simulink model "b0307"  (R2025b)
settings: Solver=ode4  StartTime=0.0  StopTime=533  FixedStep=0.001  RelTol=1e-3
values from neighbouring files (symbols this model uses):
  alpha_vector = [-8 -4 -2 0 2 3 4 5 6 8 10 12]    [aerodata.mat]    (also in airdate.m = [-8 -4 -2 0 2 3 4 5 6 8 10 12]')
  alpha_vector1 = [-4 0 4 8]    [aerodata.mat]    (also in airdate.m = [-4, 0, 4, 8])
  alpha_vector2 = [-4 0 4 8]    [aerodata.mat]    (also in airdate.m = [-4, 0, 4, 8])
  b_ref = 2.24    [init.m]
  beta_vector1 = [-8 -4 0 4 8]    [aerodata.mat]    (also in airdate.m = [-8, -4, 0, 4, 8])
  c_ref = 0.165    [init.m]
  CD_alpha = [0.0485620740363 0.0318356514345 0.0317790643102 0.0364045204537 0.0445214008185 0.0513240541996 0.0580305477533 0.0657045426134 0.0744839493029 0.0955551011208 0.133141813384 0.18014601666]    [aerodata.mat]    (also in airdate.m = alpha_matrix(1:length(alpha_vector), 3))
  CD_beta = [0.0413061898506 0.0345389961433 0.0318356514345 0.0345389961433 0.0413061898506 0.0436826 0.0385768 0.0364045204537 0.0371657170379 0.0408604078007 0.0616785 0.0590205 ... (20 elements, 5x4)]    [aerodata.mat]    (also in airdate.m = reshape(beta_matrix(:, 3), [n_beta, n_alpha1]))
  CD_ELE = [0.0367807192259 0.0308673912055 0.0306770192219 0.0329799710874 0.0376266798938 0.0362372767671 0.0347486720958 0.0364045204537 0.0395900797854 0.0493584368547 0.0520155680915 0.0546030505455 ... (20 elements, 5x4)]    [aerodata.mat]    (also in airdate.m = reshape(def_ELE_L_matrix(:, 4), [n_ele, n_alpha2]))
  CL_alpha = [-0.316928256932 -0.0246785813034 0.130283368141 0.288945629191 0.449323999783 0.525648685194 0.60297649153 0.678148219772 0.750129216407 0.872962476804 0.920788454091 0.929116005788]    [aerodata.mat]    (also in airdate.m = alpha_matrix(1:length(alpha_vector), 5))
  Cl_alpha = [-0.000640872979326 1.08116418077e-05 2.92649499784e-07 0 -0.000437066219056 -0.000762440123061 -0.000973039479867 -0.00125684277681 -0.00152984821199 -0.00187186802219 -0.00184918573213 0.00105936824418]    [aerodata.mat]    (also in airdate.m = alpha_matrix(1:length(alpha_vector), 6))
  CL_beta = [-0.0254603323809 -0.0249297140554 -0.0246785813034 -0.0249297140554 -0.0254603323809 0.27807 0.286078 0.288945629191 0.286671909097 0.27925707766 0.602944 0.604359 ... (20 elements, 5x4)]    [aerodata.mat]    (also in airdate.m = reshape(beta_matrix(:, 5), [n_beta, n_alpha1]))
  Cl_beta = [0.000236297001567 0.000139283426539 1.08116418077e-05 -0.000139283426539 -0.000236297001567 0.000738099 0.000299952 -0.000269027677603 -0.00096883985561 -0.00179948469019 0.0018278 0.000411742 ... (20 elements, 5x4)]    [aerodata.mat]    (also in airdate.m = reshape(beta_matrix(:, 6), [n_beta, n_alpha1]))
  CL_ELE = [-0.209245674304 -0.118097376915 -0.0691301102129 -0.0258480382303 0.0604619193477 0.145712419951 0.241076881119 0.288945629191 0.337037782187 0.427489906586 0.461138992576 0.556875751161 ... (20 elements, 5x4)]    [aerodata.mat]    (also in airdate.m = reshape(def_ELE_L_matrix(:, 6), [n_ele, n_alpha2]))
  Cl_ELE = [-0.0251269797289 -0.008426817179 0.000240167384607 0.00909972758991 0.0243415498089 -0.0265884432031 -0.00914521718395 -0.000269027677603 0.00845228310052 0.0248325485851 -0.027436226674 -0.00980497383292 ... (20 elements, 5x4)]    [aerodata.mat]    (also in airdate.m = reshape(def_ELE_L_matrix(:, 7), [n_ele, n_alpha2]))
  Cl_ELER = [0.0251269797289 0.008426817179 -0.000240167384607 -0.00909972758991 -0.0243415498089 0.0265884432031 0.00914521718395 0.000269027677603 -0.00845228310052 -0.0248325485851 0.027436226674 0.00980497383292 ... (20 elements, 5x4)]    [aerodata.mat]    (also in airdate.m = -Cl_ELE)
  Cm_alpha = [0.0626600725128 0.0530799370217 0.0636683163616 0.0662391704182 0.0712518097577 0.059404297375 0.0463976401398 0.0265816846325 -0.000744425674427 -0.0975303788137 -0.390110677431 -0.549514574144]    [aerodata.mat]    (also in airdate.m = alpha_matrix(1:length(alpha_vector), 7))
  Cm_beta = [0.0443576401398 0.0504624 0.0530799370217 0.0504624 0.0443576401398 0.0399653 0.0540624 0.0662391704182 0.0664956832735 0.054831924477 -0.0180401 0.0135503 ... (20 elements, 5x4)]    [aerodata.mat]    (also in airdate.m = reshape(beta_matrix(:, 7), [n_beta, n_alpha1]))
  Cm_ELE = [0.536255917663 0.147824254744 -0.0380057879786 -0.216266528425 -0.571251073338 0.641418774301 0.260817426469 0.0662391704182 -0.124486673615 -0.489660800762 0.614897515281 0.238355554417 ... (20 elements, 5x4)]    [aerodata.mat]    (also in airdate.m = reshape(def_ELE_L_matrix(:, 8), [n_ele, n_alpha2]))
  Cn_alpha = [-0.000921303455433 -0.000100429360075 -5.32721662229e-05 0 -0.000448050865233 -0.000265660085507 -0.000172455805371 -9.0297395806e-05 0.000114919609077 0.000960640598216 0.000800025371357 0.00296984280205]    [aerodata.mat]    (also in airdate.m = alpha_matrix(1:length(alpha_vector), 8))
  Cn_beta = [-0.0118929295373 -0.00644657732457 -0.000100429360075 0.00644657732457 0.0118929295373 -0.00932594 -0.00455936 -0.000185600362027 0.00379534502079 0.00738347341913 -0.00140779 -0.00161764 ... (20 elements, 5x4)]    [aerodata.mat]    (also in airdate.m = reshape(beta_matrix(:, 8), [n_beta, n_alpha1]))
  Cn_ELE = [-0.000978013358228 0.000374192483935 0.000921206928251 0.00041612460588 -0.00121710528947 -0.00219374024917 -0.000325070715732 -0.000185600362027 -8.6022941264e-05 -0.000494144283219 -0.00293821245405 -0.00054824676514 ... (20 elements, 5x4)]    [aerodata.mat]    (also in airdate.m = reshape(def_ELE_L_matrix(:, 9), [n_ele, n_alpha2]))
  Cn_ELER = [0.000978013358228 -0.000374192483935 -0.000921206928251 -0.00041612460588 0.00121710528947 0.00219374024917 0.000325070715732 0.000185600362027 8.6022941264e-05 0.000494144283219 0.00293821245405 0.00054824676514 ... (20 elements, 5x4)]    [aerodata.mat]    (also in airdate.m = -Cn_ELE)
  CY_alpha = [0.00094331940582 8.91316440807e-05 0.00163191368255 0 0.00399491029065 0.00495876756067 0.00538171092978 0.00589122371949 0.00623993707833 0.00649420059364 0.0115896523304 0.0134657730505]    [aerodata.mat]    (also in airdate.m = alpha_matrix(1:length(alpha_vector), 4))
  CY_beta = [0.0411779977966 0.0260529022214 8.91316440807e-05 -0.0260529022214 -0.0411779977966 0.0626258 0.0323129 0.00352355870293 -0.0237421290295 -0.0494841840717 0.0422501 0.0258494 ... (20 elements, 5x4)]    [aerodata.mat]    (also in airdate.m = reshape(beta_matrix(:, 4), [n_beta, n_alpha1]))
  CY_ELE = [0.00947355235179 0.0032440045221 0.000919743913066 3.31170671791e-05 -0.00246607912146 0.00984559930618 0.00470476147172 0.00352355870293 0.00144187166173 -0.00241087659802 0.0116316527742 0.00697261934365 ... (20 elements, 5x4)]    [aerodata.mat]    (also in airdate.m = reshape(def_ELE_L_matrix(:, 5), [n_ele, n_alpha2]))
  def_ELE_L_vector = [-15 -5 0 5 15]    [aerodata.mat]    (also in airdate.m = [-15, -5, 0, 5, 15])
  delta_max = 15    [init.m]
  fly_pt = [0 397.202504295 825.49541327 510 4564.45331975 4885.85117615 4860 4885.85117615 4899.67498335 5610.29789652 5624.12170371 5880 ... (135 elements, 27x5)]    [baseline_fly_plan.mat]    (also in debug_replay_flyphase.m = evalin('base','fly_pt'); dubins_path_planning.m = dubins.filter_waypoints(fly_pt); fly_planfjy.mat; make_orbit_plan.m = dubins.filter_waypoints(fly_pt))
  g = 9.8    [Astar.m]    (also in dubins_path_planning.m; init.m; make_orbit_plan.m; make_route_plan.m)
  I = [I_x -I_xy -I_xz ... (first row only)    [init.m]
  I_inv = inv(I)    [init.m]
  kal = (wn^2-a_24(3))/(2*zeta*wn)    [controller.m]
  ki = 0.1*kphi    (= 0.75)    [controller.m]
  kn = (-2.2*wn^2*g)/(Tr*(wn^2+a_24(3))*Vc*Z_al)    [controller.m]
  kp = 2*zeta2*wn2/N_delatr_bar    [controller.m]
  kphi = wn2/2/zeta2    (= 7.5)    [controller.m]
  kq = -(2*zeta*wn) / a_25    [controller.m]
  mass = 27.1    [init.m]
  pitch_max = 30    [init.m]
  psi_0 = 0 * (pi/180)    (= 0)    [init.m]
  psi_t = 0    [Astar.m]    (also in init.m)
  roll_max = 30*pi/180    (= 0.523598775598)    [Astar.m]    (also in dubins_path_planning.m = 0.261799387799; init.m = 30)
  S_ref = 0.7    [init.m]
  theta_0 = 30 * (pi/180)    (= 0.523598775598)    [init.m]
  theta_t = 0    [Astar.m]    (also in init.m)
  u_0 = Vc_0*cos(beta_0)*cos(alpha_0)    [init.m]
  v_0 = Vc_0*sin(beta_0)    [init.m]
  V_t = 0    [Astar.m]    (also in init.m)
  Vc = 34    [Astar.m]    (also in dubins_path_planning.m; init.m; make_orbit_plan.m; make_route_plan.m)
  w_0 = Vc_0*cos(beta_0)*sin(alpha_0)    [init.m]
  W_down = 0    [init.m]
  W_east = 0    [init.m]
  W_north = 0    [init.m]
  xt0 = 6500    [Astar.m]    (also in init.m)
  yt0 = 9000    [Astar.m]    (also in init.m)
  Z_al = (CD_alpha(10)+CL_al)*(q_0*S_ref/(mass*Vc))    [controller.m]
  zt0 = 0    [Astar.m]    (also in init.m)
undefined symbols (not defined in the file or in its folder): beta_vector0
libraries: matrix_library x2, simulink x1, aerolibatmos2 x1, slpidlib x1
(part 2 of 2)

== system b0307/气动力和气动力矩/气动力/侧力 ==
  q_p1 : Inport
  beta1 : Inport  Port=2
  alpha1 : Inport  Port=3
  delta_l : Inport  Port=4
  delta_r : Inport  Port=5
  Add : Sum  Inputs=-+
  Add1 : Sum  Inputs=+-
  Add2 : Sum  Inputs=+-
  Add3 : Sum  Inputs=+-
  Add4 : Sum
  Add5 : Sum  Inputs=++++
  CY_alpha : Lookup_n-D  NumberOfTableDimensions=1  BreakpointsForDimension1=alpha_vector  BreakpointsForDimension2=beta_vector0  BreakpointsForDimension3=[5, 7]  Table=CY_alpha  InternalRulePriority=Speed  RndMeth=Simplest
  CY_alpha0 : Lookup_n-D  NumberOfTableDimensions=1  BreakpointsForDimension1=alpha_vector  BreakpointsForDimension2=beta_vector0  BreakpointsForDimension3=[5, 7]  Table=CY_alpha  InternalRulePriority=Speed  RndMeth=Simplest
  CY_beta : Lookup_n-D  BreakpointsForDimension1=beta_vector1  BreakpointsForDimension2=alpha_vector1  BreakpointsForDimension3=[5, 7]  Table=CY_beta  InternalRulePriority=Speed  RndMeth=Simplest
      settings: InputPortMap=u0,u1
  CY_beta0 : Lookup_n-D  BreakpointsForDimension1=beta_vector1  BreakpointsForDimension2=alpha_vector1  BreakpointsForDimension3=[5, 7]  Table=CY_beta  InternalRulePriority=Speed  RndMeth=Simplest
      settings: InputPortMap=u0,u1
  CY_delta_l : Lookup_n-D  BreakpointsForDimension1=def_ELE_L_vector  BreakpointsForDimension2=alpha_vector2  BreakpointsForDimension3=[5, 7]  Table=CY_ELE  InternalRulePriority=Speed  RndMeth=Simplest
      settings: InputPortMap=u0,u1
  CY_delta_l0 : Lookup_n-D  BreakpointsForDimension1=def_ELE_L_vector  BreakpointsForDimension2=alpha_vector2  BreakpointsForDimension3=[5, 7]  Table=CY_ELE  InternalRulePriority=Speed  RndMeth=Simplest
      settings: InputPortMap=u0,u1
  CY_delta_r : Lookup_n-D  BreakpointsForDimension1=def_ELE_L_vector  BreakpointsForDimension2=alpha_vector2  BreakpointsForDimension3=[5, 7]  Table=CY_ELE  InternalRulePriority=Speed  RndMeth=Simplest
      settings: InputPortMap=u0,u1
  CY_delta_r0 : Lookup_n-D  BreakpointsForDimension1=def_ELE_L_vector  BreakpointsForDimension2=alpha_vector2  BreakpointsForDimension3=[5, 7]  Table=CY_ELE  InternalRulePriority=Speed  RndMeth=Simplest
      settings: InputPortMap=u0,u1
  Constant : Constant  Value=0
  Constant1 : Constant  Value=0
  Constant7 : Constant  Value=S_ref
  Product : Product  Inputs=3
  Saturation : Saturate  UpperLimit=8  LowerLimit=-4
  侧力Y : Outport
  wires:
  Add3/1 -> Add4/2
  delta_l/1 -> CY_delta_l/1
  CY_delta_l0/1 -> Add2/2
  Add1/1 -> Add5/3
  CY_alpha/1 -> Add/2
  q_p1/1 -> Product/1
  Add4/1 -> Add5/4
  Constant7/1 -> Product/3
  Add5/1 -> Product/2
  Add2/1 -> Add4/1
  CY_delta_r/1 -> Add3/1
  CY_alpha0/1 -> Add/1, Add5/1
  Add/1 -> Add5/2
  Product/1 -> 侧力Y/1
  CY_beta0/1 -> Add1/2
  Constant1/1 -> CY_delta_r0/1, CY_delta_l0/1
  CY_delta_l/1 -> Add2/1
  Constant/1 -> CY_beta0/1, CY_alpha0/1
  CY_delta_r0/1 -> Add3/2
  delta_r/1 -> CY_delta_r/1
  alpha1/1 -> Saturation/1, CY_alpha/1
  beta1/1 -> CY_beta/1
  CY_beta/1 -> Add1/1
  Saturation/1 -> CY_beta0/2, CY_delta_l/2, CY_delta_l0/2, CY_delta_r0/2, CY_delta_r/2, CY_beta/2

== system b0307/气动力和气动力矩/气动力/升力 ==
  q_p : Inport
  beta : Inport  Port=2
  alpha : Inport  Port=3
  delta_l : Inport  Port=4
  delta_r : Inport  Port=5
  Add : Sum  Inputs=-+
  Add1 : Sum  Inputs=+-
  Add2 : Sum  Inputs=+-
  Add3 : Sum  Inputs=+-
  Add4 : Sum
  Add5 : Sum  Inputs=++++
  CL_alpha : Lookup_n-D  NumberOfTableDimensions=1  BreakpointsForDimension1=alpha_vector  Table=CL_alpha  ExtrapMethod=Clip  UseLastTableValue=on  InternalRulePriority=Speed  RndMeth=Simplest
  CL_beta : Lookup_n-D  BreakpointsForDimension1=beta_vector1  BreakpointsForDimension2=alpha_vector1  BreakpointsForDimension3=[5, 7]  Table=CL_beta  InternalRulePriority=Speed  RndMeth=Simplest
      settings: InputPortMap=u0,u1
  CL_beta0 : Lookup_n-D  BreakpointsForDimension1=beta_vector1  BreakpointsForDimension2=alpha_vector1  BreakpointsForDimension3=[5, 7]  Table=CL_beta  InternalRulePriority=Speed  RndMeth=Simplest
      settings: InputPortMap=u0,u1
  CL_delta_l : Lookup_n-D  BreakpointsForDimension1=def_ELE_L_vector  BreakpointsForDimension2=alpha_vector2  BreakpointsForDimension3=[5, 7]  Table=CL_ELE  InternalRulePriority=Speed  RndMeth=Simplest
      settings: InputPortMap=u0,u1
  CL_delta_l0 : Lookup_n-D  BreakpointsForDimension1=def_ELE_L_vector  BreakpointsForDimension2=alpha_vector2  BreakpointsForDimension3=[5, 7]  Table=CL_ELE  InternalRulePriority=Speed  RndMeth=Simplest
      settings: InputPortMap=u0,u1
  CL_delta_r : Lookup_n-D  BreakpointsForDimension1=def_ELE_L_vector  BreakpointsForDimension2=alpha_vector2  BreakpointsForDimension3=[5, 7]  Table=CL_ELE  InternalRulePriority=Speed  RndMeth=Simplest
      settings: InputPortMap=u0,u1
  CL_delta_r0 : Lookup_n-D  BreakpointsForDimension1=def_ELE_L_vector  BreakpointsForDimension2=alpha_vector2  BreakpointsForDimension3=[5, 7]  Table=CL_ELE  InternalRulePriority=Speed  RndMeth=Simplest
      settings: InputPortMap=u0,u1
  Constant : Constant  Value=0
  Constant1 : Constant  Value=0
  Constant7 : Constant  Value=S_ref
  Product : Product  Inputs=3
  Saturation : Saturate  UpperLimit=8  LowerLimit=-4
  cL0 : Lookup_n-D  NumberOfTableDimensions=1  BreakpointsForDimension1=alpha_vector  Table=CL_alpha  ExtrapMethod=Clip  UseLastTableValue=on  InternalRulePriority=Speed  RndMeth=Simplest
  升力L : Outport
  wires:
  alpha/1 -> Saturation/1, CL_alpha/1
  CL_alpha/1 -> Add/2
  cL0/1 -> Add/1, Add5/1
  Constant/1 -> CL_beta0/1, cL0/1
  beta/1 -> CL_beta/1
  CL_beta0/1 -> Add1/2
  CL_beta/1 -> Add1/1
  delta_r/1 -> CL_delta_r/1
  delta_l/1 -> CL_delta_l/1
  Constant1/1 -> CL_delta_r0/1, CL_delta_l0/1
  CL_delta_l/1 -> Add2/1
  CL_delta_l0/1 -> Add2/2
  CL_delta_r/1 -> Add3/1
  CL_delta_r0/1 -> Add3/2
  Add2/1 -> Add4/1
  Add3/1 -> Add4/2
  Add4/1 -> Add5/4
  Add1/1 -> Add5/3
  Add/1 -> Add5/2
  Add5/1 -> Product/2
  q_p/1 -> Product/1
  Product/1 -> 升力L/1
  Constant7/1 -> Product/3
  Saturation/1 -> CL_beta0/2, CL_delta_r0/2, CL_delta_r/2, CL_delta_l0/2, CL_delta_l/2, CL_beta/2

== system b0307/气动力和气动力矩/气动力/阻力 ==
  q_p1 : Inport
  beta1 : Inport  Port=2
  alpha1 : Inport  Port=3
  delta_l : Inport  Port=4
  delta_r : Inport  Port=5
  Add : Sum  Inputs=-+
  Add1 : Sum  Inputs=+-
  Add2 : Sum  Inputs=+-
  Add3 : Sum  Inputs=+-
  Add4 : Sum
  Add5 : Sum  Inputs=++++
  CD_alpha : Lookup_n-D  NumberOfTableDimensions=1  BreakpointsForDimension1=alpha_vector  Table=CD_alpha  ExtrapMethod=Clip  UseLastTableValue=on  InternalRulePriority=Speed  RndMeth=Simplest
  CD_beta : Lookup_n-D  BreakpointsForDimension1=beta_vector1  BreakpointsForDimension2=alpha_vector1  BreakpointsForDimension3=[5, 7]  Table=CD_beta  InternalRulePriority=Speed  RndMeth=Simplest
      settings: InputPortMap=u0,u1
  CD_beta0 : Lookup_n-D  BreakpointsForDimension1=beta_vector1  BreakpointsForDimension2=alpha_vector1  BreakpointsForDimension3=[5, 7]  Table=CD_beta  InternalRulePriority=Speed  RndMeth=Simplest
      settings: InputPortMap=u0,u1
  CD_delta_l : Lookup_n-D  BreakpointsForDimension1=def_ELE_L_vector  BreakpointsForDimension2=alpha_vector2  BreakpointsForDimension3=[5, 7]  Table=CD_ELE  InternalRulePriority=Speed  RndMeth=Simplest
      settings: InputPortMap=u0,u1
  CD_delta_l0 : Lookup_n-D  BreakpointsForDimension1=def_ELE_L_vector  BreakpointsForDimension2=alpha_vector2  BreakpointsForDimension3=[5, 7]  Table=CD_ELE  InternalRulePriority=Speed  RndMeth=Simplest
      settings: InputPortMap=u0,u1
  CD_delta_r : Lookup_n-D  BreakpointsForDimension1=def_ELE_L_vector  BreakpointsForDimension2=alpha_vector2  BreakpointsForDimension3=[5, 7]  Table=CD_ELE  InternalRulePriority=Speed  RndMeth=Simplest
      settings: InputPortMap=u0,u1
  CD_delta_r0 : Lookup_n-D  BreakpointsForDimension1=def_ELE_L_vector  BreakpointsForDimension2=alpha_vector2  BreakpointsForDimension3=[5, 7]  Table=CD_ELE  InternalRulePriority=Speed  RndMeth=Simplest
      settings: InputPortMap=u0,u1
  Constant : Constant  Value=0
  Constant1 : Constant  Value=0
  Constant7 : Constant  Value=S_ref
  Product : Product  Inputs=3
  Saturation : Saturate  UpperLimit=8  LowerLimit=-4
  cD0 : Lookup_n-D  NumberOfTableDimensions=1  BreakpointsForDimension1=alpha_vector  Table=CD_alpha  ExtrapMethod=Clip  UseLastTableValue=on  InternalRulePriority=Speed  RndMeth=Simplest
  阻力L : Outport
  wires:
  Add3/1 -> Add4/2
  delta_l/1 -> CD_delta_l/1
  CD_delta_l0/1 -> Add2/2
  Add1/1 -> Add5/3
  CD_alpha/1 -> Add/2
  q_p1/1 -> Product/1
  Add4/1 -> Add5/4
  Constant7/1 -> Product/3
  Add5/1 -> Product/2
  Add2/1 -> Add4/1
  CD_delta_r/1 -> Add3/1
  cD0/1 -> Add/1, Add5/1
  Add/1 -> Add5/2
  Product/1 -> 阻力L/1
  CD_beta0/1 -> Add1/2
  Constant1/1 -> CD_delta_r0/1, CD_delta_l0/1
  CD_delta_l/1 -> Add2/1
  Constant/1 -> CD_beta0/1, cD0/1
  CD_delta_r0/1 -> Add3/2
  delta_r/1 -> CD_delta_r/1
  alpha1/1 -> Saturation/1, CD_alpha/1
  beta1/1 -> CD_beta/1
  CD_beta/1 -> Add1/1
  Saturation/1 -> CD_delta_l/2, CD_delta_l0/2, CD_delta_r0/2, CD_delta_r/2, CD_beta0/2, CD_beta/2

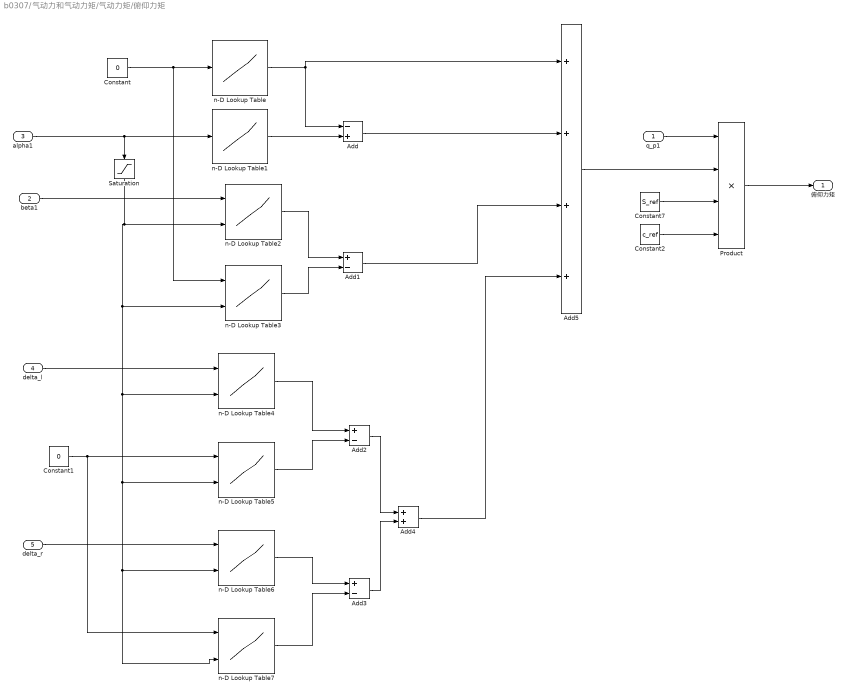
== system b0307/气动力和气动力矩/气动力矩/俯仰力矩 ==
  q_p1 : Inport
  beta1 : Inport  Port=2
  alpha1 : Inport  Port=3
  delta_l : Inport  Port=4
  delta_r : Inport  Port=5
  Add : Sum  Inputs=-+
  Add1 : Sum  Inputs=+-
  Add2 : Sum  Inputs=+-
  Add3 : Sum  Inputs=+-
  Add4 : Sum
  Add5 : Sum  Inputs=++++
  Constant : Constant  Value=0
  Constant1 : Constant  Value=0
  Constant2 : Constant  Value=c_ref
  Constant7 : Constant  Value=S_ref
  Product : Product  Inputs=4
  Saturation : Saturate  UpperLimit=8  LowerLimit=-4
  n-D Lookup Table : Lookup_n-D  NumberOfTableDimensions=1  BreakpointsForDimension1=alpha_vector  BreakpointsForDimension3=[5, 7]  Table=Cm_alpha  InternalRulePriority=Speed  RndMeth=Simplest
  n-D Lookup Table1 : Lookup_n-D  NumberOfTableDimensions=1  BreakpointsForDimension1=alpha_vector  BreakpointsForDimension3=[5, 7]  Table=Cm_alpha  InternalRulePriority=Speed  RndMeth=Simplest
  n-D Lookup Table2 : Lookup_n-D  BreakpointsForDimension1=beta_vector1  BreakpointsForDimension2=alpha_vector1  BreakpointsForDimension3=[5, 7]  Table=Cm_beta  InternalRulePriority=Speed  RndMeth=Simplest
      settings: InputPortMap=u0,u1
  n-D Lookup Table3 : Lookup_n-D  BreakpointsForDimension1=beta_vector1  BreakpointsForDimension2=alpha_vector1  BreakpointsForDimension3=[5, 7]  Table=Cm_beta  InternalRulePriority=Speed  RndMeth=Simplest
      settings: InputPortMap=u0,u1
  n-D Lookup Table{4..7} (4 alike) : Lookup_n-D  BreakpointsForDimension1=def_ELE_L_vector  BreakpointsForDimension2=alpha_vector2  BreakpointsForDimension3=[5, 7]  Table=Cm_ELE  InternalRulePriority=Speed  RndMeth=Simplest
      settings: InputPortMap=u0,u1
  俯仰力矩 : Outport
  wires:
  Add3/1 -> Add4/2
  delta_l/1 -> n-D Lookup Table4/1
  n-D Lookup Table5/1 -> Add2/2
  Add1/1 -> Add5/3
  n-D Lookup Table1/1 -> Add/2
  q_p1/1 -> Product/1
  Add4/1 -> Add5/4
  Constant7/1 -> Product/3
  Add5/1 -> Product/2
  Add2/1 -> Add4/1
  n-D Lookup Table6/1 -> Add3/1
  n-D Lookup Table/1 -> Add/1, Add5/1
  Add/1 -> Add5/2
  Product/1 -> 俯仰力矩/1
  n-D Lookup Table3/1 -> Add1/2
  Constant1/1 -> n-D Lookup Table7/1, n-D Lookup Table5/1
  n-D Lookup Table4/1 -> Add2/1
  Constant/1 -> n-D Lookup Table3/1, n-D Lookup Table/1
  n-D Lookup Table7/1 -> Add3/2
  delta_r/1 -> n-D Lookup Table6/1
  alpha1/1 -> Saturation/1, n-D Lookup Table1/1
  beta1/1 -> n-D Lookup Table2/1
  n-D Lookup Table2/1 -> Add1/1
  Constant2/1 -> Product/4
  Saturation/1 -> n-D Lookup Table3/2, n-D Lookup Table4/2, n-D Lookup Table5/2, n-D Lookup Table7/2, n-D Lookup Table6/2, n-D Lookup Table2/2

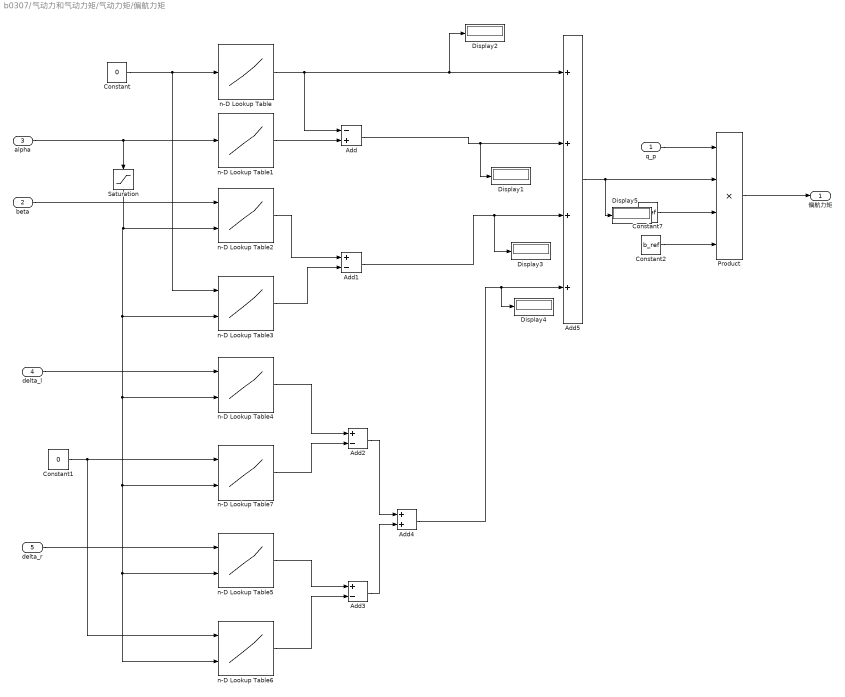
== system b0307/气动力和气动力矩/气动力矩/偏航力矩 ==
  q_p : Inport
  beta : Inport  Port=2
  alpha : Inport  Port=3
  delta_l : Inport  Port=4
  delta_r : Inport  Port=5
  Add : Sum  Inputs=-+
  Add1 : Sum  Inputs=+-
  Add2 : Sum  Inputs=+-
  Add3 : Sum  Inputs=+-
  Add4 : Sum
  Add5 : Sum  Inputs=++++
  Constant : Constant  Value=0
  Constant1 : Constant  Value=0
  Constant2 : Constant  Value=b_ref
  Constant7 : Constant  Value=S_ref
  Display{1..5} (5 alike) : Display
  Product : Product  Inputs=4
  Saturation : Saturate  UpperLimit=8  LowerLimit=-4
  n-D Lookup Table : Lookup_n-D  NumberOfTableDimensions=1  BreakpointsForDimension1=alpha_vector  BreakpointsForDimension3=[5, 7]  Table=Cn_alpha  InternalRulePriority=Speed  RndMeth=Simplest
  n-D Lookup Table1 : Lookup_n-D  NumberOfTableDimensions=1  BreakpointsForDimension1=alpha_vector  BreakpointsForDimension3=[5, 7]  Table=Cn_alpha  InternalRulePriority=Speed  RndMeth=Simplest
  n-D Lookup Table2 : Lookup_n-D  BreakpointsForDimension1=beta_vector1  BreakpointsForDimension2=alpha_vector1  BreakpointsForDimension3=[5, 7]  Table=Cn_beta  InternalRulePriority=Speed  RndMeth=Simplest
      settings: InputPortMap=u0,u1
  n-D Lookup Table3 : Lookup_n-D  BreakpointsForDimension1=beta_vector1  BreakpointsForDimension2=alpha_vector1  BreakpointsForDimension3=[5, 7]  Table=Cn_beta  InternalRulePriority=Speed  RndMeth=Simplest
      settings: InputPortMap=u0,u1
  n-D Lookup Table4 : Lookup_n-D  BreakpointsForDimension1=def_ELE_L_vector  BreakpointsForDimension2=alpha_vector2  BreakpointsForDimension3=[5, 7]  Table=Cn_ELE  InternalRulePriority=Speed  RndMeth=Simplest
      settings: InputPortMap=u0,u1
  n-D Lookup Table5 : Lookup_n-D  BreakpointsForDimension1=def_ELE_L_vector  BreakpointsForDimension2=alpha_vector2  BreakpointsForDimension3=[5, 7]  Table=Cn_ELER  InternalRulePriority=Speed  RndMeth=Simplest
      settings: InputPortMap=u0,u1
  n-D Lookup Table6 : Lookup_n-D  BreakpointsForDimension1=def_ELE_L_vector  BreakpointsForDimension2=alpha_vector2  BreakpointsForDimension3=[5, 7]  Table=Cn_ELER  InternalRulePriority=Speed  RndMeth=Simplest
      settings: InputPortMap=u0,u1
  n-D Lookup Table7 : Lookup_n-D  BreakpointsForDimension1=def_ELE_L_vector  BreakpointsForDimension2=alpha_vector2  BreakpointsForDimension3=[5, 7]  Table=Cn_ELE  InternalRulePriority=Speed  RndMeth=Simplest
      settings: InputPortMap=u0,u1
  偏航力矩 : Outport
  wires:
  alpha/1 -> Saturation/1, n-D Lookup Table1/1
  n-D Lookup Table1/1 -> Add/2
  n-D Lookup Table/1 -> Add/1, Display2/1, Add5/1
  Constant/1 -> n-D Lookup Table3/1, n-D Lookup Table/1
  beta/1 -> n-D Lookup Table2/1
  n-D Lookup Table3/1 -> Add1/2
  n-D Lookup Table2/1 -> Add1/1
  delta_r/1 -> n-D Lookup Table5/1
  delta_l/1 -> n-D Lookup Table4/1
  Constant1/1 -> n-D Lookup Table6/1, n-D Lookup Table7/1
  n-D Lookup Table4/1 -> Add2/1
  n-D Lookup Table7/1 -> Add2/2
  n-D Lookup Table5/1 -> Add3/1
  n-D Lookup Table6/1 -> Add3/2
  Add2/1 -> Add4/1
  Add3/1 -> Add4/2
  Add4/1 -> Display4/1, Add5/4
  Add1/1 -> Display3/1, Add5/3
  Add/1 -> Display1/1, Add5/2
  Add5/1 -> Display5/1, Product/2
  q_p/1 -> Product/1
  Product/1 -> 偏航力矩/1
  Constant7/1 -> Product/3
  Constant2/1 -> Product/4
  Saturation/1 -> n-D Lookup Table3/2, n-D Lookup Table4/2, n-D Lookup Table7/2, n-D Lookup Table6/2, n-D Lookup Table5/2, n-D Lookup Table2/2

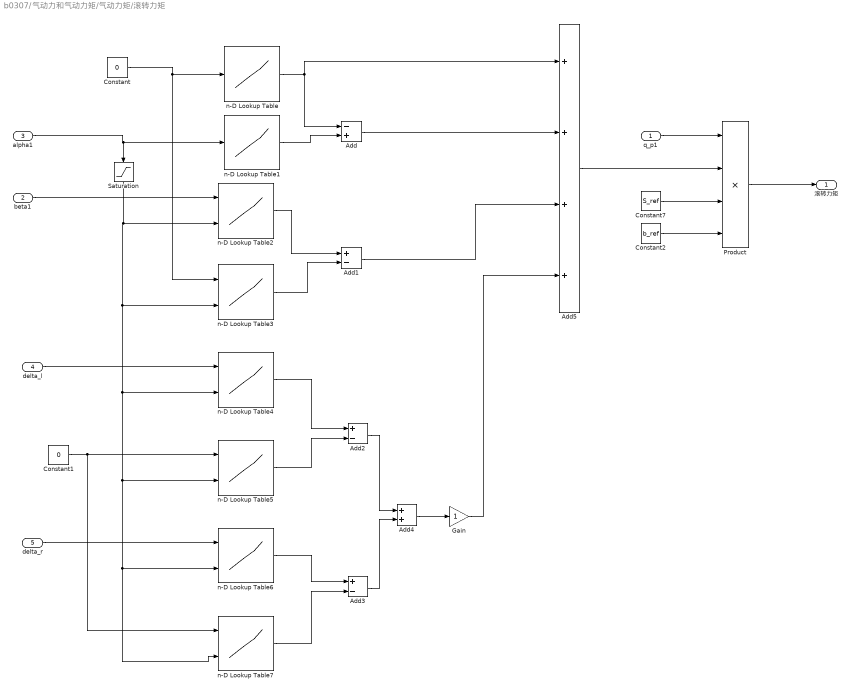
== system b0307/气动力和气动力矩/气动力矩/滚转力矩 ==
  q_p1 : Inport
  beta1 : Inport  Port=2
  alpha1 : Inport  Port=3
  delta_l : Inport  Port=4
  delta_r : Inport  Port=5
  Add : Sum  Inputs=-+
  Add1 : Sum  Inputs=+-
  Add2 : Sum  Inputs=+-
  Add3 : Sum  Inputs=+-
  Add4 : Sum
  Add5 : Sum  Inputs=++++
  Constant : Constant  Value=0
  Constant1 : Constant  Value=0
  Constant2 : Constant  Value=b_ref
  Constant7 : Constant  Value=S_ref
  Gain : Gain
  Product : Product  Inputs=4
  Saturation : Saturate  UpperLimit=8  LowerLimit=-4
  n-D Lookup Table : Lookup_n-D  NumberOfTableDimensions=1  BreakpointsForDimension1=alpha_vector  BreakpointsForDimension3=[5, 7]  Table=Cl_alpha  InternalRulePriority=Speed  RndMeth=Simplest
  n-D Lookup Table1 : Lookup_n-D  NumberOfTableDimensions=1  BreakpointsForDimension1=alpha_vector  BreakpointsForDimension3=[5, 7]  Table=Cl_alpha  InternalRulePriority=Speed  RndMeth=Simplest
  n-D Lookup Table2 : Lookup_n-D  BreakpointsForDimension1=beta_vector1  BreakpointsForDimension2=alpha_vector1  BreakpointsForDimension3=[5, 7]  Table=Cl_beta  InternalRulePriority=Speed  RndMeth=Simplest
      settings: InputPortMap=u0,u1
  n-D Lookup Table3 : Lookup_n-D  BreakpointsForDimension1=beta_vector1  BreakpointsForDimension2=alpha_vector1  BreakpointsForDimension3=[5, 7]  Table=Cl_beta  InternalRulePriority=Speed  RndMeth=Simplest
      settings: InputPortMap=u0,u1
  n-D Lookup Table4 : Lookup_n-D  BreakpointsForDimension1=def_ELE_L_vector  BreakpointsForDimension2=alpha_vector2  BreakpointsForDimension3=[5, 7]  Table=Cl_ELE  InternalRulePriority=Speed  RndMeth=Simplest
      settings: InputPortMap=u0,u1
  n-D Lookup Table5 : Lookup_n-D  BreakpointsForDimension1=def_ELE_L_vector  BreakpointsForDimension2=alpha_vector2  BreakpointsForDimension3=[5, 7]  Table=Cl_ELE  InternalRulePriority=Speed  RndMeth=Simplest
      settings: InputPortMap=u0,u1
  n-D Lookup Table6 : Lookup_n-D  BreakpointsForDimension1=def_ELE_L_vector  BreakpointsForDimension2=alpha_vector2  BreakpointsForDimension3=[5, 7]  Table=Cl_ELER  InternalRulePriority=Speed  RndMeth=Simplest
      settings: InputPortMap=u0,u1
  n-D Lookup Table7 : Lookup_n-D  BreakpointsForDimension1=def_ELE_L_vector  BreakpointsForDimension2=alpha_vector2  BreakpointsForDimension3=[5, 7]  Table=Cl_ELER  InternalRulePriority=Speed  RndMeth=Simplest
      settings: InputPortMap=u0,u1
  滚转力矩 : Outport
  wires:
  Add3/1 -> Add4/2
  delta_l/1 -> n-D Lookup Table4/1
  n-D Lookup Table5/1 -> Add2/2
  Add1/1 -> Add5/3
  n-D Lookup Table1/1 -> Add/2
  q_p1/1 -> Product/1
  Add4/1 -> Gain/1
  Constant7/1 -> Product/3
  Add5/1 -> Product/2
  Add2/1 -> Add4/1
  n-D Lookup Table6/1 -> Add3/1
  n-D Lookup Table/1 -> Add5/1, Add/1
  Add/1 -> Add5/2
  Product/1 -> 滚转力矩/1
  n-D Lookup Table3/1 -> Add1/2
  Constant1/1 -> n-D Lookup Table7/1, n-D Lookup Table5/1
  n-D Lookup Table4/1 -> Add2/1
  Constant/1 -> n-D Lookup Table3/1, n-D Lookup Table/1
  n-D Lookup Table7/1 -> Add3/2
  delta_r/1 -> n-D Lookup Table6/1
  alpha1/1 -> Saturation/1, n-D Lookup Table1/1
  beta1/1 -> n-D Lookup Table2/1
  n-D Lookup Table2/1 -> Add1/1
  Constant2/1 -> Product/4
  Saturation/1 -> n-D Lookup Table3/2, n-D Lookup Table4/2, n-D Lookup Table5/2, n-D Lookup Table7/2, n-D Lookup Table6/2, n-D Lookup Table2/2
  Gain/1 -> Add5/4

== system b0307/制导系统/制导系统/巡航段制导/航向制导回路 ==
  速度 : Inport
  侧偏 : Inport  Port=2
  Abs1 : Abs  SaturateOnIntegerOverflow=off
  Abs3 : Abs  SaturateOnIntegerOverflow=off
  Constant : Constant  Value=0
  Constant3 : Constant  Value=1.8
  MinMax : MinMax  Inputs=2
  Product2 : Product
  Saturation2 : Saturate  UpperLimit=40  LowerLimit=-40
  Saturation3 : Saturate  UpperLimit=6  LowerLimit=-6
  Scope2 : Scope  NumInputPorts=2
      settings: ActiveDisplayYMinimum=-92.743821036367819  ActiveDisplayYMaximum=91.709558289732186  DataLoggingVariableName=ScopeData5
  Scope5 : Scope
      settings: ActiveDisplayYMinimum=-0.28125000000000006  ActiveDisplayYMaximum=0.28125000000000006  DataLoggingVariableName=ScopeData3
  Scope8 : Scope
      settings: ActiveDisplayYMinimum=-1.252400949515843  ActiveDisplayYMaximum=0.71434371328293278  DataLoggingVariableName=ScopeData36
  Sign : Signum
  Sum3 : Sum  Inputs=|+-
  Sum4 : Sum  Inputs=|+-
  kdy : Gain  Gain=0.02
  kdy_dot : Gain  Gain=0.2
  Nyc : Outport
  wires:
  侧偏/1 -> Sum3/2, Scope2/2
  Constant/1 -> Scope2/1, Sum3/1
  速度/1 -> Saturation3/1
  Sum3/1 -> Saturation2/1
  Saturation3/1 -> kdy_dot/1
  Saturation2/1 -> kdy/1
  kdy/1 -> Sum4/1
  kdy_dot/1 -> Sum4/2
  Abs1/1 -> MinMax/1
  Sign/1 -> Product2/1
  Constant3/1 -> Abs3/1
  MinMax/1 -> Product2/2
  Abs3/1 -> MinMax/2
  Product2/1 -> Nyc/1, Scope5/1
  Sum4/1 -> Sign/1, Abs1/1, Scope8/1

== system b0307/制导系统/制导系统/巡航段制导/高度控制回路 ==
  速度 : Inport
  Abs1 : Abs  SaturateOnIntegerOverflow=off
  Constant2 : Constant  Value=3
  Gain1 : Gain  Gain=-1
  MinMax : MinMax  Inputs=2
  Product2 : Product
  Saturation : Saturate  UpperLimit=40  LowerLimit=-40
  Saturation1 : Saturate  UpperLimit=10  LowerLimit=-10
  Scope1 : Scope  NumInputPorts=2
      settings: ActiveDisplayYMinimum=-37.499999999999993  ActiveDisplayYMaximum=337.5  DataLoggingVariableName=ScopeData4
  Scope4 : Scope
      settings: ActiveDisplayYMinimum=-3.3669517762061467  ActiveDisplayYMaximum=0.30256598585532024  DataLoggingVariableName=ScopeData24
  Selector : Selector  InputPortWidth=3  IndexOptions=Index vector (dialog)  Indices=[3]  OutputSizes=1
  Selector1 : Selector  InputPortWidth=5  IndexOptions=Index vector (dialog)  Indices=3  OutputSizes=1
  Sign : Signum
  Sum : Sum  Inputs=-+
  Sum1 : Sum  Inputs=|++
  Sum2 : Sum
  Trigonometric Function : Trigonometry  Operator=cos
  kh : Gain  Gain=0.04
  khd : Gain  Gain=0.12
  Nzc : Outport
  wires:
  Gain1/1 -> Abs1/1, Sign/1
  Selector/1 -> Saturation1/1
  Saturation/1 -> kh/1
  kh/1 -> Sum1/1
  [h_g] -> Sum/1, Scope1/1
  khd/1 -> Sum1/2
  Sum2/1 -> Gain1/1
  Saturation1/1 -> khd/1
  Sum/1 -> Saturation/1
  Sign/1 -> Product2/1
  Sum1/1 -> Sum2/2
  Constant2/1 -> MinMax/2
  MinMax/1 -> Product2/2
  [theta] -> Trigonometric Function/1
  Product2/1 -> Nzc/1, Scope4/1
  Trigonometric Function/1 -> Sum2/1
  Abs1/1 -> MinMax/1
  速度/1 -> Selector/1
  Selector1/1 -> Scope1/2, Sum/2
  [next_pt] -> Selector1/1

== matlab function b0307/航路跟踪/MATLAB Function ==
  settings: updateMethod=DISCRETE  sampleTime=0.001
  data: dy input; fly_phase output; fly_type output; prev_pt output size=[1, 5]; next_pt output size=[1, 5]; DTG input; time input; fly_pt input; coc_pt output size=[1, 5]; xyz_g input
function [fly_phase, fly_type, prev_pt, next_pt, coc_pt] = fly_phase(dy, DTG, time, fly_pt, xyz_g)

xyz_g = xyz_g(:)';  % 统一转为行向量 [x, y, z]

persistent fly_phase_temp fly_type_temp coc_pt_temp prev_pt_temp next_pt_temp arc_entered
if isempty(fly_phase_temp)
    fly_phase_temp = 1;
    arc_entered = false;
    % 初始化数据提取（调用下面定义的子函数）
    [fly_type_temp, prev_pt_temp, next_pt_temp, coc_pt_temp, fly_phase_temp] = ...
        update_segment_data(fly_pt, fly_phase_temp);
end

has_crossed = false;

if time > 0.1 % 稍微给一点初始化时间
    if fly_type_temp == 1
        % --- 直线段切换逻辑 ---
        seg_vec = next_pt_temp(1:3) - prev_pt_temp(1:3);
        seg_len = norm(seg_vec);
        if seg_len > 1e-3
            seg_dir = seg_vec / seg_len;
            curr_vec = xyz_g - prev_pt_temp(1:3);
            along = dot(curr_vec, seg_dir);
            % 只要投影距离超过总长，就切换
            has_crossed = (along >= seg_len);
        else
            has_crossed = true; % 长度太短直接跳过
        end
        arc_entered = false;

    elseif fly_type_temp == 2
        % --- 圆弧段切换逻辑 ---
        x0 = coc_pt_temp(1); y0 = coc_pt_temp(2);
        radius = coc_pt_temp(5);
        dir_type = prev_pt_temp(5); % 1=右转(CW), 2=左转(CCW)
        
        dist_to_center = norm(xyz_g(1:2) - [x0, y0]);
        
        % 判断是否进入有效圆弧跟踪区（防止切入前的误判）
        if ~arc_entered
            % 距离圆心误差在30%以内或距离目标点较近时，锁定圆弧逻辑
            if abs(dist_to_center - radius) < radius * 0.3 || DTG < 50
                arc_entered = true;
            end
        end

        if arc_entered
            theta_entry = atan2(prev_pt_temp(2) - y0, prev_pt_temp(1) - x0);
            theta_exit  = atan2(next_pt_temp(2) - y0, next_pt_temp(1) - x0);
            theta_curr  = atan2(xyz_g(2) - y0, xyz_g(1) - x0);

            if dir_type == 1 % 右转，顺时针，角度递减
                total_sweep = mod(theta_entry - theta_exit, 2*pi);
                sweep = mod(theta_entry - theta_curr, 2*pi);
            else % 左转，逆时针，角度递增
                total_sweep = mod(theta_exit - theta_entry, 2*pi);
                sweep = mod(theta_curr - theta_entry, 2*pi);
            end
            % 扫过角度达到总角度则切换
            has_crossed = (sweep >= total_sweep - 0.01); % 留一点裕量
        end
    end
end

% --- 执行切换逻辑 ---
if has_crossed
    % 指针先加1
    fly_phase_temp = fly_phase_temp + 1;
    
    % [核心修复] 自动跳过重复点或极近点
    while fly_phase_temp + 1 < size(fly_pt, 1)
        dist_to_next = norm(fly_pt(fly_phase_temp, 1:2) - fly_pt(fly_phase_temp+1, 1:2));
        % 如果两行点坐标太近（< 0.5m），说明是冗余点，直接继续跳
        if dist_to_next < 0.5
            fly_phase_temp = fly_phase_temp + 1;
        else
            break;
        end
    end
    
    % 更新段数据
    if fly_phase_temp + 1 <= size(fly_pt, 1)
        [fly_type_temp, prev_pt_temp, next_pt_temp, coc_pt_temp, fly_phase_temp] = ...
            update_segment_data(fly_pt, fly_phase_temp);
        arc_entered = false;
    end
end

% 输出赋值
prev_pt = prev_pt_temp;
next_pt = next_pt_temp;
coc_pt = coc_pt_temp;
fly_type = fly_type_temp;
fly_phase = fly_phase_temp;

end

% --- 辅助函数：根据当前索引提取下一段的完整信息 ---
function [type, p_pt, n_pt, c_pt, new_idx] = update_segment_data(fly_pt, idx)
    new_idx = idx;
    p_pt = fly_pt(new_idx, :);
    type = p_pt(4);
    
    % 默认目标点是下一行
    n_pt = fly_pt(new_idx + 1, :);
    c_pt = [0 0 0 1 0]; % 直线段默认圆心
    
    % 如果当前段是圆弧，且下一行(new_idx+1)是圆心定义行
    % 判断标准：Type=2 且 Info(第5列) 不是 1 或 2 (而是半径)
    if type == 2
        cand_n_pt = fly_pt(new_idx + 1, :);
        if cand_n_pt(4) == 2 && cand_n_pt(5) ~= 1 && cand_n_pt(5) ~= 2
            % 确认 new_idx+1 是圆心行
            c_pt = cand_n_pt;
            % 真正的目标点应该是圆心行的下一行
            if new_idx + 2 <= size(fly_pt, 1)
                new_idx = new_idx + 1; % 跳过圆心行
                n_pt = fly_pt(new_idx + 1, :);
            end
        end
    end
end

== matlab function b0307/动力学和运动学/平动动力学/V2B1 ==
  data: alpha input; R_bwind output; beta input
function R_bwind = wind2body(alpha, beta)
T1 = [cos(alpha), 0, sin(alpha);
       0, 1, 0;
       -sin(alpha), 0, cos(alpha)];
T2 = [cos(beta), sin(beta), 0;
       -sin(beta), cos(beta), 0;
       0, 0, 1];
R_wind_b = T2*T1;
R_bwind = R_wind_b';

== matlab function b0307/动力学和运动学/平动动力学/G2B ==
  data: phi input; R_bg output; theta input; psi input
function R_bg = ground2body(phi, theta, psi)
T1 = [cos(psi), sin(psi), 0;
     -sin(psi), cos(psi), 0;
      0, 0, 1];
T2 = [cos(theta), 0, -sin(theta);
       0, 1, 0;
      sin(theta), 0, cos(theta)];
T3 = [1, 0, 0;
      0, cos(phi), sin(phi);
      0, -sin(phi), cos(phi)];
R_bg = T3 * T2 * T1;

== matlab function b0307/动力学和运动学/位置积分/MATLAB Function ==
  data: R_bg output; phi input; theta input; psi input
function R_bg = ground2body(phi, theta, psi)
T1 = [cos(psi), sin(psi), 0;
     -sin(psi), cos(psi), 0;
      0, 0, 1];
T2 = [cos(theta), 0, -sin(theta);
       0, 1, 0;
      sin(theta), 0, cos(theta)];
T3 = [1, 0, 0;
      0, cos(phi), sin(phi);
      0, -sin(phi), cos(phi)];
R_bg = T3 * T2 * T1;

== matlab function b0307/动力学和运动学/攻角侧滑角计算 ==
  data: u input; V output; v input; w input; alpha output; beta output; q_p output; rho input
function [V, alpha, beta, q_p] = airdata(u, v, w,rho )
%% 1. 速度大小
V = sqrt(u*u + v*v + w*w);

%% 2. 数值保护（防止除0）
V_safe = max(V, 1e-6);

%% 3. 攻角 alpha
alpha = atan2(w, u);

%% 4. 侧滑角 beta
x = v / V_safe;
beta = asin(x);
%% 5. 动压
q_p = 0.5*rho*V*V;

end

== matlab function b0307/制导系统/制导系统/BTT/btt ==
  data: nz_b output; phi_c output; nz_c input; ny_c input
function [nz_b, phi_c] = BTT(nz_c ,ny_c)
n_combine = sign(nz_c)*sqrt(nz_c^2+ny_c^2);

if abs(n_combine)<.1
    if n_combine > 0
        n_temp = .1;
    else
        n_temp = -.1;
    end
else
    n_temp = n_combine;
end
nz_b = n_temp;
phi_c = -asin(ny_c/nz_b);

== matlab function b0307/航路跟踪/MATLAB Function1 ==
  settings: updateMethod=DISCRETE  sampleTime=0.001
  data: fly_type input; prev_pt input; next_pt input; coc_pt input; xyz_g input; Vxyz_g input; dy output; dy_dot output; DTG output
function [dy, dy_dot, DTG] = dy_dydot_subsystem(fly_type, prev_pt, next_pt, coc_pt, xyz_g, Vxyz_g)

    if fly_type == 1
        [dy, dy_dot, DTG] = line_calculation(prev_pt, next_pt, xyz_g, Vxyz_g);
    elseif fly_type == 2
        [dy, dy_dot] = dy_dydot_circle(coc_pt, xyz_g, prev_pt, Vxyz_g);
        DTG = dtg_circle(next_pt, xyz_g, coc_pt);
    else
        [dy, dy_dot, DTG] = line_calculation(prev_pt, next_pt, xyz_g, Vxyz_g);
    end

end

function [dy_line, dy_dot_line, DTG_line] = line_calculation(prev_pt, next_pt, current_pt, Vxyz_g)
%line_calculation 直线段侧偏距、侧偏距变化率、剩余距离计算

    % 提取坐标
    x1 = prev_pt(1); y1 = prev_pt(2);
    x2 = next_pt(1); y2 = next_pt(2);
    x  = current_pt(1); y = current_pt(2);
    vx = Vxyz_g(1); vy = Vxyz_g(2);

    % === 计算路径方向角 ===
    dx = x2 - x1;
    dy = y2 - y1;

    if dx > 0
        true_psi = atan2(dy, dx);
    elseif dx < 0
        true_psi = pi - atan2(dy, abs(dx));
    else
        if dy > 0
            true_psi = pi/2;
        elseif dy < 0
            true_psi = 3*pi/2;
        else
            true_psi = 0;
        end
    end

    % === 构建旋转矩阵并转换到路径坐标系 ===
    % 路径坐标系: 第1轴为侧偏方向, 第2轴为沿航方向
    c = cos(true_psi);
    s = sin(true_psi);
    T = [c, -s; s, c];              % 旋转矩阵

    V_prev_next = T * [y2 - y1; x2 - x1];   % 路径在路径坐标系中 = [0; |P|]
    V_prev_curr = T * [y - y1;  x - x1];    % 当前位置在路径坐标系中 = [dy; along]

    % === 侧偏距 dy  ===

    dy_line = V_prev_curr(1);

    % === 剩余距离 DTG ===
    norm_next = norm(V_prev_next);
    if norm_next > 1e-10
        L_temp = dot(V_prev_next, V_prev_curr) / norm_next;  % 沿航迹投影
        DTG_line = norm_next - L_temp;
    else
        DTG_line = 0;
    end

    % === 侧偏距变化率 dy_dot ===

    dy_dot_line = -vx * s + vy * c;

end
function DTG = dtg_circle(next_pt, current_pt, coc_pt)
%dtg_circle 圆弧段剩余弧长计算
    % 提取坐标
    x_cur  = current_pt(1); y_cur  = current_pt(2);
    x_next = next_pt(1);    y_next = next_pt(2);
    x0 = coc_pt(1);         y0 = coc_pt(2);
    radius = coc_pt(5);

    % 当前位置->圆心向量、目标点->圆心向量
    O_cur = [x_cur - x0,  y_cur - y0];
    O_nex = [x_next - x0, y_next - y0];

    % 两向量夹角 (防止acos数值越界)
    cos_angle = dot(O_cur, O_nex) / (norm(O_cur) * norm(O_nex) + eps);
    cos_angle = min(max(cos_angle, -1), 1);

    % 弧长 = 半径 x 夹角
    DTG = radius * acos(cos_angle);

end
function [dy_circle, dy_dot_circle] = dy_dydot_circle(coc_pt, current_pt, prev_pt, Vxyz_g)

    % 提取数据
    x0 = coc_pt(1);      y0 = coc_pt(2);
    radius = coc_pt(5);
    x_cur = current_pt(1); y_cur = current_pt(2);
    vx = Vxyz_g(1); vy = Vxyz_g(2);

    dir_type = prev_pt(5);   % 1=右转, 2=左转

    % 当前位置到圆心的距离
    L_O = norm([x_cur - x0, y_cur - y0]);

    % 径向向量 (圆心->飞机) 和径向单位向量
    if L_O > 1e-10
        radial_unit = [x_cur - x0, y_cur - y0] / L_O;
    else
        radial_unit = [0, 0];
    end

    % 速度在径向方向的投影: cos_angle2 = dot(v, radial) / (|v| * L)
    v_norm = sqrt(vx^2 + vy^2);
    if v_norm > 1e-10
        cos_angle2 = (vx * radial_unit(1) + vy * radial_unit(2)) / v_norm;
    else
        cos_angle2 = 0;
    end

    % 根据转向类型计算 dy 和 dy_dot
    if dir_type == 1        % 右转: 圆内为正(偏右)
        dy_circle = -radius + L_O;
        dy_dot_circle = v_norm * cos_angle2;   % 径向向外速度(朝向路径)
    elseif dir_type == 2    % 左转: 圆外为正(偏右)
        dy_circle = -L_O + radius;
        dy_dot_circle = -v_norm * cos_angle2;  % 径向向内速度(朝向路径)
    else
        dy_circle = 0;
        dy_dot_circle = 0;
    end

end

== matlab function b0307/动力学和运动学/风场计算 ==
  data: u input; u_a output; v input; w input; phi input; theta input; psi input; W_n input; W_e input; W_d input; v_a output; w_a output
function [u_a, v_a, w_a] = wind_comp(u, v, w, phi, theta, psi, W_n, W_e, W_d)
% 风速从 NED 系转到体轴系，地速减去风速得到空速
cphi = cos(phi); sphi = sin(phi);
cth  = cos(theta); sth  = sin(theta);
cpsi = cos(psi);   spsi = sin(psi);
% NED -> Body DCM 旋转
wind_x =  cth*cpsi*W_n + cth*spsi*W_e - sth*W_d;
wind_y = (sphi*sth*cpsi - cphi*spsi)*W_n + (sphi*sth*spsi + cphi*cpsi)*W_e + sphi*cth*W_d;
wind_z = (cphi*sth*cpsi + sphi*spsi)*W_n + (cphi*sth*spsi - sphi*cpsi)*W_e + cphi*cth*W_d;
% 空速 = 地速 - 风速
u_a = u - wind_x;
v_a = v - wind_y;
w_a = w - wind_z;
end
